simulink model "Controllo_Ottimo_LQG"  (R2023b)
settings: Solver=VariableStepAuto  StartTime=0.0  StopTime=50  RelTol=1e-3
undefined symbols (not defined in the file): A, A_Kal, B, B_Kal, C, C_Kal, D, D_Kal, Fi, Fr, Tc
libraries: simulink x2
settings Model: Creator=emman  LastModifiedBy=emman

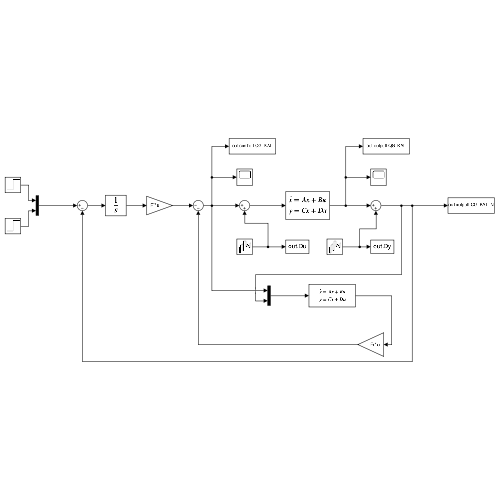
[thumbnail: Simulink's stored preview of the top-level diagram]
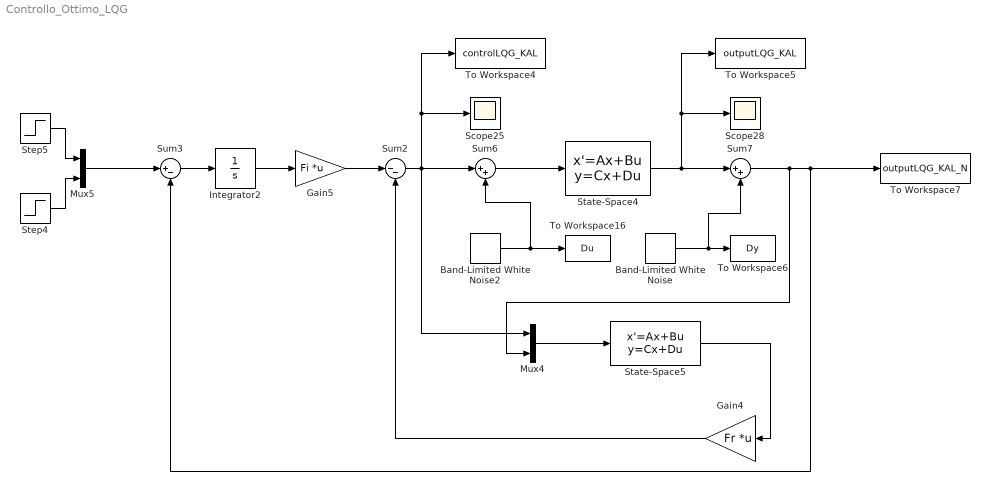
== system Controllo_Ottimo_LQG ==
  Band-Limited White Noise : simulink/Sources/Band-Limited White Noise  Cov=NoisePower  Ts=Tc  seed=[23341]
  Band-Limited White Noise2 : simulink/Sources/Band-Limited White Noise  Cov=Qnoise  Ts=Tc  seed=[23341]
  Gain4 : Gain  Gain=Fr  Multiplication=Matrix(K*u)
  Gain5 : Gain  Gain=Fi  Multiplication=Matrix(K*u)
  Integrator2 : Integrator
  Mux4 : Mux  Inputs=2
  Mux5 : Mux  Inputs=2
  Scope25 : Scope
  Scope28 : Scope
  State-Space4 : StateSpace  A=A  B=B  C=C  D=D  InitialCondition=0  ParameterTunability=Unconstrained
  State-Space5 : StateSpace  A=A_Kal  B=B_Kal  C=C_Kal  D=D_Kal  InitialCondition=0
  Step4 : Step  Time=0  After=2.5  SampleTime=0
  Step5 : Step  Time=0  After=2  SampleTime=0
  Sum2 : Sum  Inputs=|--
  Sum3 : Sum  Inputs=|+-
  Sum6 : Sum  Inputs=|++
  Sum7 : Sum  Inputs=|++
  To Workspace16 : ToWorkspace  VariableName=Du  SaveFormat=Structure With Time  SampleTime=-1
  To Workspace4 : ToWorkspace  VariableName=controlLQG_KAL  SaveFormat=Structure With Time  SampleTime=-1
  To Workspace5 : ToWorkspace  VariableName=outputLQG_KAL  SaveFormat=Structure With Time  SampleTime=-1
  To Workspace6 : ToWorkspace  VariableName=Dy  SaveFormat=Structure With Time  SampleTime=-1
  To Workspace7 : ToWorkspace  VariableName=outputLQG_KAL_N  SaveFormat=Structure With Time  SampleTime=-1
  wires:
  Mux4/1 -> State-Space5/1
  Band-Limited White Noise2/1 -> Sum6/2, To Workspace16/1
  Band-Limited White Noise/1 -> Sum7/2, To Workspace6/1
  State-Space5/1 -> Gain4/1
  State-Space4/1 -> Scope28/1, To Workspace5/1, Sum7/1
  Step5/1 -> Mux5/1
  Sum7/1 -> To Workspace7/1, Sum3/2, Mux4/2
  Integrator2/1 -> Gain5/1
  Gain5/1 -> Sum2/1
  Gain4/1 -> Sum2/2
  Sum6/1 -> State-Space4/1
  Sum3/1 -> Integrator2/1
  Step4/1 -> Mux5/2
  Mux5/1 -> Sum3/1
  Sum2/1 -> Scope25/1, To Workspace4/1, Mux4/1, Sum6/1
